simulink model "compute_next_state_2019a"  (R2019a)
settings: Solver=FixedStepAuto  StartTime=0.0  StopTime=10.0  FixedStep=1/400  RelTol=1e-3
settings Model: Creator=Julius  LastModifiedBy=brandlju
settings OptimizationCC: LocalBlockOutputs=off
settings DebuggingCC: SFMachineParentedDataDiag=error
settings RTWCC: SystemTargetFile=TwinCAT.tlc  GenCodeOnly=on  MakeCommand=make_tct  TemplateMakefile=tct_msbuild.tmf  Description=TwinCAT Target  GenerateReport=on  TargetLang=C++
settings STFCustomTargetCC: TargetLangStandard=C++03 (ISO)  CompOptLevelCompliant=on  MATLABClassNameForMDSCustomization=Simulink.SoftwareTarget.TargetSpecificTriggerConfigurationBase  SystemTargetFile=TwinCAT.tlc

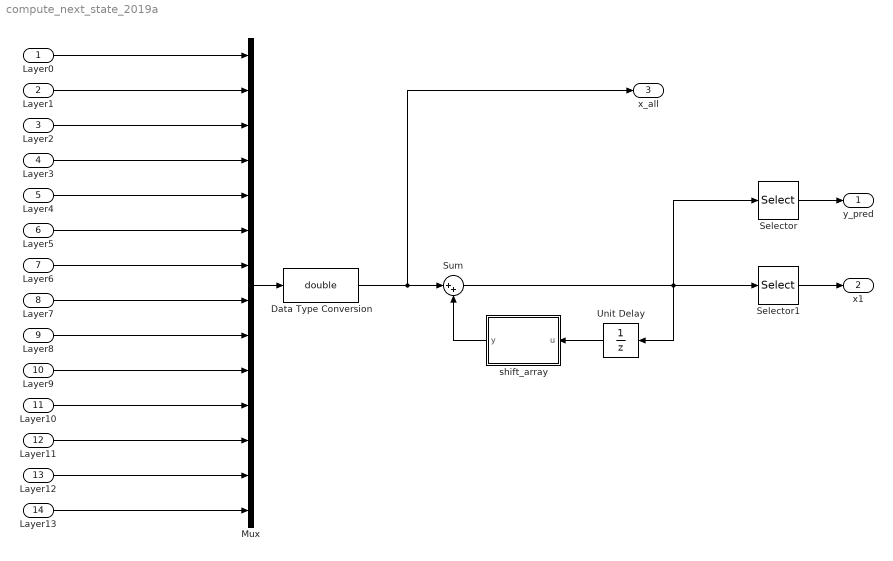
== system compute_next_state_2019a ==
  Layer0 : Inport  OutDataTypeStr=single  PortDimensions=1
  Layer1 : Inport  Port=2  OutDataTypeStr=single  PortDimensions=1
  Layer2 : Inport  Port=3  OutDataTypeStr=single  PortDimensions=1
  Layer3 : Inport  Port=4  OutDataTypeStr=single  PortDimensions=1
  Layer4 : Inport  Port=5  OutDataTypeStr=single  PortDimensions=1
  Layer5 : Inport  Port=6  OutDataTypeStr=single  PortDimensions=1
  Layer6 : Inport  Port=7  OutDataTypeStr=single  PortDimensions=1
  Layer7 : Inport  Port=8  OutDataTypeStr=single  PortDimensions=1
  Layer8 : Inport  Port=9  OutDataTypeStr=single  PortDimensions=1
  Layer9 : Inport  Port=10  OutDataTypeStr=single  PortDimensions=1
  Layer10 : Inport  Port=11  OutDataTypeStr=single  PortDimensions=1
  Layer11 : Inport  Port=12  OutDataTypeStr=single  PortDimensions=1
  Layer12 : Inport  Port=13  OutDataTypeStr=single  PortDimensions=1
  Layer13 : Inport  Port=14  OutDataTypeStr=single  PortDimensions=1
  Data Type Conversion : DataTypeConversion  OutDataTypeStr=double
  Mux : Mux  Inputs=14
  Selector : Selector  InputPortWidth=14  IndexOptions=Index vector (dialog)  Indices=[1]  OutputSizes=1
  Selector1 : Selector  InputPortWidth=14  IndexOptions=Index vector (dialog)  Indices=[2]  OutputSizes=1
  Sum : Sum  Inputs=|++
  Unit Delay : UnitDelay  InitialCondition=zeros(14, 1)  SampleTime=-1  HasFrameUpgradeWarning=on
  shift_array : MATLAB Function  TreatAsAtomicUnit=on
  y_pred : Outport  OutDataTypeStr=double  VectorParamsAs1DForOutWhenUnconnected=on
  x1 : Outport  Port=2  OutDataTypeStr=double  PortDimensions=1  VectorParamsAs1DForOutWhenUnconnected=on
  x_all : Outport  Port=3  OutDataTypeStr=double  PortDimensions=14  VectorParamsAs1DForOutWhenUnconnected=on
  wires:
  Mux/1 -> Data Type Conversion/1
  Unit Delay/1 -> shift_array/1(u)
  shift_array/1(y) -> Sum/2
  Selector/1 -> y_pred/1
  Sum/1 -> Selector1/1, Selector/1, Unit Delay/1
  Layer1/1 -> Mux/2
  Layer2/1 -> Mux/3
  Layer3/1 -> Mux/4
  Layer4/1 -> Mux/5
  Layer5/1 -> Mux/6
  Layer6/1 -> Mux/7
  Layer7/1 -> Mux/8
  Layer8/1 -> Mux/9
  Layer9/1 -> Mux/10
  Layer10/1 -> Mux/11
  Layer11/1 -> Mux/12
  Layer12/1 -> Mux/13
  Layer13/1 -> Mux/14
  Selector1/1 -> x1/1
  Data Type Conversion/1 -> x_all/1, Sum/1
  Layer0/1 -> Mux/1

== matlab function compute_next_state_2019a/shift_array ==
  data: u input; y output
function y = fcn(u)
y = [u(2:end, 1); 0];
